simulink model "VCU_TDN"  (R2020a)
settings: Solver=FixedStepDiscrete  StartTime=0.0  StopTime=10.0  FixedStep=0.001  RelTol=1e-3  EnableMultiTasking=on
InitFcn:
  | EcoCoder_PreCheckLic();
undefined symbols (not defined in the file or in its folder): h, km
libraries: CoderSF_BSW_Libs x187, simulink x9, SF_CanService_Libs x1
(part 2 of 2)

== system VCU_TDN/Code/Initialization/Disabling the inverter ==
  Constant : Constant  Value=hex2dec('51')  OutDataTypeStr=uint8
  Constant1 : Constant  Value=hex2dec('0004')  OutDataTypeStr=uint16
  Pack Signals To CAN Data : CoderSF_BSW_Libs/CAN/Pack Signals To CAN Data  Signal="{{'REG_ID'  'Data1'},[0 8],[8 16],{'uint8'  'uint16'},{'Intel' 'Intel'}}"
  Send CAN Data : CoderSF_BSW_Libs/CAN/Send CAN Data  channel=CAN_A  txlen=3  txid=hex2dec('201')  frametype=Standard(11-bit ID)  showerror=off
  wires:
  Constant/1 -> Pack Signals To CAN Data/1
  Pack Signals To CAN Data/1 -> Send CAN Data/1
  Constant1/1 -> Pack Signals To CAN Data/2

== system VCU_TDN/Code/Ready to drive/Activate Ready to drive ==
  Trigger : TriggerPort  VariantControl=Variant
  Constant{,1,3..4} (4 alike) : Constant  OutDataTypeStr=boolean
  Enabling the inverter : Subsystem
  FRG/RUN : CoderSF_BSW_Libs/Digital I//O/Switch Output  channel=LSO07
  RFE : CoderSF_BSW_Libs/Digital I//O/Switch Output  channel=LSO06
  Ready to drive LED : CoderSF_BSW_Libs/Digital I//O/Switch Output  channel=LSO08
  Ready to drive sound : CoderSF_BSW_Libs/Digital I//O/Switch Output  channel=LSO10
  wires:
  Constant1/1 -> FRG/RUN/1
  Constant/1 -> RFE/1
  Constant3/1 -> Ready to drive LED/1
  Constant4/1 -> Ready to drive sound/1

== system VCU_TDN/Code/Ready to drive/Deactivate Ready to drive ==
  Trigger : TriggerPort  VariantControl=Variant
  Constant : Constant  Value=0  OutDataTypeStr=boolean
  Constant1 : Constant  Value=0  OutDataTypeStr=boolean
  Constant3 : Constant  Value=0  OutDataTypeStr=boolean
  Disabling the inverter : Subsystem
  FRG/RUN : CoderSF_BSW_Libs/Digital I//O/Switch Output  channel=LSO07
  RFE : CoderSF_BSW_Libs/Digital I//O/Switch Output  channel=LSO06
  Ready to drive LED : CoderSF_BSW_Libs/Digital I//O/Switch Output  channel=LSO08
  wires:
  Constant1/1 -> FRG/RUN/1
  Constant/1 -> RFE/1
  Constant3/1 -> Ready to drive LED/1

== system VCU_TDN/Code/Ready to drive/Stop RTD sound ==
  Trigger : TriggerPort  VariantControl=Variant
  Constant4 : Constant  Value=0  OutDataTypeStr=boolean
  Ready to drive sound : CoderSF_BSW_Libs/Digital I//O/Switch Output  channel=LSO10
  wires:
  Constant4/1 -> Ready to drive sound/1

== system VCU_TDN/Code/Receiving data/BMS ==

== system VCU_TDN/Code/Receiving data/Battery temperature sensors ==

== system VCU_TDN/Code/Receiving data/Inverter ==
  Data saving : Subsystem  TreatAsAtomicUnit=on
  Read CAN Message : SF_CanService_Libs/Read CAN Message  typeCAN=Connected  channel=CAN_A  mEn=off  msgInfo=can  msgIterm=INV_VCU  msgItermStore=INV_VCU  valid=on  stale=off  motoBit=off  setSignalName=off  flgCustomMonitorVariableRules=on  defineSignalName=off  prefixSignal='rx'  flgValTest=off  flgNoFixed=on  tSample=Task_L10ms  modeCode=Parameterless
  wires:
  Read CAN Message/1 -> Data saving/Trigger
  Read CAN Message/3 -> Data saving/2(Data)
  Read CAN Message/2 -> Data saving/1(RegID)

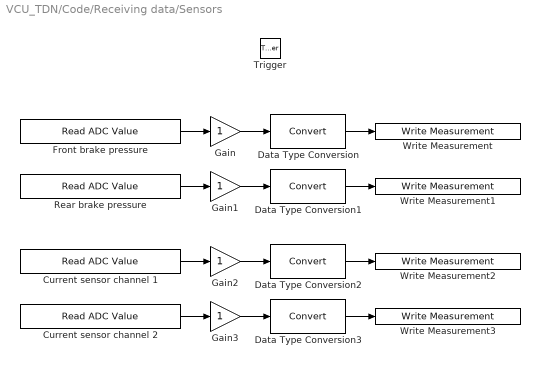
== system VCU_TDN/Code/Receiving data/Sensors ==
  Trigger : TriggerPort  TriggerType=function-call  VariantControl=Variant  PortDimensions=1
  Current sensor channel 1 : CoderSF_BSW_Libs/ADC/Read ADC Value  channel=15
  Current sensor channel 2 : CoderSF_BSW_Libs/ADC/Read ADC Value  channel=17
  Data Type Conversion{,1..3} (4 alike) : DataTypeConversion
  Front brake pressure : CoderSF_BSW_Libs/ADC/Read ADC Value  channel=8
  Gain{,1..3} (4 alike) : Gain
  Rear brake pressure : CoderSF_BSW_Libs/ADC/Read ADC Value  channel=12
  Write Measurement : CoderSF_BSW_Libs/Calibration & Measurement/Write Measurement  variable_name=FR_BRK_PRESSURE  variable_value=0  variable_type=single  numD=1  unitStr=bar  descStr=""
      settings: AttributesFormatString=type:%<variable_type> Dimensions:%<numD>
  Write Measurement1 : CoderSF_BSW_Libs/Calibration & Measurement/Write Measurement  variable_name=RR_BRAKE_PRESSURE  variable_value=0  variable_type=single  numD=1  unitStr=bar  descStr=""
      settings: AttributesFormatString=type:%<variable_type> Dimensions:%<numD>
  Write Measurement2 : CoderSF_BSW_Libs/Calibration & Measurement/Write Measurement  variable_name=CURRENT_CH_1  variable_value=0  variable_type=int16  numD=1  unitStr=A  descStr=""
      settings: AttributesFormatString=type:%<variable_type> Dimensions:%<numD>
  Write Measurement3 : CoderSF_BSW_Libs/Calibration & Measurement/Write Measurement  variable_name=CURRENT_CH_2  variable_value=0  variable_type=int16  numD=1  unitStr=A  descStr=""
      settings: AttributesFormatString=type:%<variable_type> Dimensions:%<numD>
  wires:
  Current sensor channel 2/1 -> Gain3/1
  Current sensor channel 1/1 -> Gain2/1
  Rear brake pressure/1 -> Gain1/1
  Front brake pressure/1 -> Gain/1
  Data Type Conversion/1 -> Write Measurement/1
  Data Type Conversion3/1 -> Write Measurement3/1
  Gain2/1 -> Data Type Conversion2/1
  Data Type Conversion2/1 -> Write Measurement2/1
  Gain1/1 -> Data Type Conversion1/1
  Data Type Conversion1/1 -> Write Measurement1/1
  Gain/1 -> Data Type Conversion/1
  Gain3/1 -> Data Type Conversion3/1

== system VCU_TDN/Code/Ready to drive/Activate Ready to drive/Enabling the inverter ==
  Constant : Constant  Value=hex2dec('51')  OutDataTypeStr=uint8
  Constant1 : Constant  Value=hex2dec('0000')  OutDataTypeStr=uint16
  Pack Signals To CAN Data : CoderSF_BSW_Libs/CAN/Pack Signals To CAN Data  Signal="{{'REG_ID'  'Data1'},[0 8],[8 16],{'uint8'  'uint16'},{'Intel' 'Intel'}}"
  Send CAN Data : CoderSF_BSW_Libs/CAN/Send CAN Data  channel=CAN_A  txlen=3  txid=hex2dec('201')  frametype=Standard(11-bit ID)  showerror=off
  wires:
  Constant/1 -> Pack Signals To CAN Data/1
  Pack Signals To CAN Data/1 -> Send CAN Data/1
  Constant1/1 -> Pack Signals To CAN Data/2

== system VCU_TDN/Code/Ready to drive/Deactivate Ready to drive/Disabling the inverter ==
  Constant : Constant  Value=hex2dec('51')  OutDataTypeStr=uint8
  Constant1 : Constant  Value=hex2dec('0004')  OutDataTypeStr=uint16
  Pack Signals To CAN Data : CoderSF_BSW_Libs/CAN/Pack Signals To CAN Data  Signal="{{'REG_ID'  'Data1'},[0 8],[8 16],{'uint8'  'uint16'},{'Intel' 'Intel'}}"
  Send CAN Data : CoderSF_BSW_Libs/CAN/Send CAN Data  channel=CAN_A  txlen=3  txid=hex2dec('201')  frametype=Standard(11-bit ID)  showerror=off
  wires:
  Constant/1 -> Pack Signals To CAN Data/1
  Pack Signals To CAN Data/1 -> Send CAN Data/1
  Constant1/1 -> Pack Signals To CAN Data/2

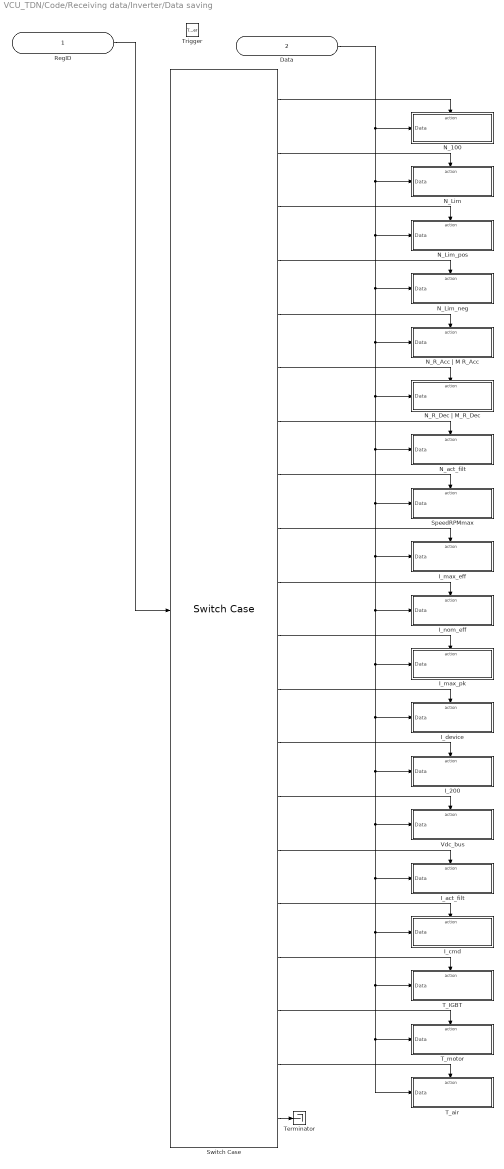
== system VCU_TDN/Code/Receiving data/Inverter/Data saving ==
  RegID : Inport
  Data : Inport  Port=2
  Trigger : TriggerPort  VariantControl=Variant
  I_200 : Subsystem  TreatAsAtomicUnit=on
  I_act_filt : Subsystem  TreatAsAtomicUnit=on
  I_cmd : Subsystem  TreatAsAtomicUnit=on
  I_device : Subsystem  TreatAsAtomicUnit=on
  I_max_eff : Subsystem  TreatAsAtomicUnit=on
  I_max_pk : Subsystem  TreatAsAtomicUnit=on
  I_nom_eff : Subsystem  TreatAsAtomicUnit=on
  N_100 : Subsystem  TreatAsAtomicUnit=on
  N_Lim : Subsystem  TreatAsAtomicUnit=on
  N_Lim_neg : Subsystem  TreatAsAtomicUnit=on
  N_Lim_pos : Subsystem  TreatAsAtomicUnit=on
  N_R_Acc | M R_Acc : Subsystem  TreatAsAtomicUnit=on
  N_R_Dec | M_R_Dec : Subsystem  TreatAsAtomicUnit=on
  N_act_filt : Subsystem  TreatAsAtomicUnit=on
  SpeedRPMmax : Subsystem  TreatAsAtomicUnit=on
  Switch Case : SwitchCase  CaseConditions={0xc8,0x34,0x3f,0x3e,0x35,0xed,0xce,0xa8,0x4d,0x4e,0xc4,0xc6,0xd9,0xeb,0x5f,0x26,0x4a,0x49,0x4b}
  T_IGBT : Subsystem  TreatAsAtomicUnit=on
  T_air : Subsystem  TreatAsAtomicUnit=on
  T_motor : Subsystem  TreatAsAtomicUnit=on
  Terminator : Terminator
  Vdc_bus : Subsystem  TreatAsAtomicUnit=on
  wires:
  RegID/1 -> Switch Case/1
  Switch Case/20 -> Terminator/1
  Switch Case/1 -> N_100/Action
  Switch Case/2 -> N_Lim/Action
  Switch Case/3 -> N_Lim_pos/Action
  Switch Case/4 -> N_Lim_neg/Action
  Switch Case/5 -> N_R_Acc | M R_Acc/Action
  Switch Case/6 -> N_R_Dec | M_R_Dec/Action
  Switch Case/7 -> N_act_filt/Action
  Switch Case/8 -> SpeedRPMmax/Action
  Switch Case/9 -> I_max_eff/Action
  Switch Case/10 -> I_nom_eff/Action
  Switch Case/11 -> I_max_pk/Action
  Switch Case/12 -> I_device/Action
  Switch Case/13 -> I_200/Action
  Switch Case/14 -> Vdc_bus/Action
  Switch Case/15 -> I_act_filt/Action
  Switch Case/16 -> I_cmd/Action
  Switch Case/17 -> T_IGBT/Action
  Switch Case/18 -> T_motor/Action
  Switch Case/19 -> T_air/Action
  Data/1 -> T_air/1(Data), T_motor/1(Data), T_IGBT/1(Data), I_cmd/1(Data), I_act_filt/1(Data), Vdc_bus/1(Data), I_200/1(Data), I_device/1(Data), I_max_pk/1(Data), I_nom_eff/1(Data), I_max_eff/1(Data), SpeedRPMmax/1(Data), N_act_filt/1(Data), N_R_Dec | M_R_Dec/1(Data), N_R_Acc | M R_Acc/1(Data), N_Lim_neg/1(Data), N_Lim_pos/1(Data), N_Lim/1(Data), N_100/1(Data)

== system VCU_TDN/Code/Receiving data/Inverter/Data saving/I_200 ==
  Data : Inport
  Action Port : ActionPort  ActionPortLabel=case [ 217 ]:
  Data Type Conversion : DataTypeConversion
  Write NVM : CoderSF_BSW_Libs/Non-volatile Memory Blocks/Write NVM  variable_name=nvmI_200  flgDef=on  variable_value=0  variable_type=int16  variable_numD=1  unitStr=""  descStr=""  EcoCoderBlockID=N001_NVMVDEF
      settings: AttributesFormatString=value:%<variable_value> type:%<variable_type> D:%<variable_numD>
  Write and Read Measurement : CoderSF_BSW_Libs/Calibration & Measurement/Write and Read Measurement  variable_name=I_200  variable_value=0  variable_type=int16  numD=1  unitStr=""  descStr=""
      settings: AttributesFormatString=type:%<variable_type> Dimensions:%<numD>
  wires:
  Data Type Conversion/1 -> Write and Read Measurement/1
  Data/1 -> Data Type Conversion/1
  Write and Read Measurement/1 -> Write NVM/1  "I_200"

== system VCU_TDN/Code/Receiving data/Inverter/Data saving/I_act_filt ==
  Data : Inport
  Action Port : ActionPort  ActionPortLabel=case [ 95 ]:
  Data Type Conversion : DataTypeConversion
  Write NVM : CoderSF_BSW_Libs/Non-volatile Memory Blocks/Write NVM  variable_name=nvmI_act_filt  flgDef=on  variable_value=0  variable_type=int16  variable_numD=1  unitStr=""  descStr=""  EcoCoderBlockID=N001_NVMVDEF
      settings: AttributesFormatString=value:%<variable_value> type:%<variable_type> D:%<variable_numD>
  Write and Read Measurement : CoderSF_BSW_Libs/Calibration & Measurement/Write and Read Measurement  variable_name=I_act_filt  variable_value=0  variable_type=int16  numD=1  unitStr=""  descStr=""
      settings: AttributesFormatString=type:%<variable_type> Dimensions:%<numD>
  wires:
  Data Type Conversion/1 -> Write and Read Measurement/1
  Data/1 -> Data Type Conversion/1
  Write and Read Measurement/1 -> Write NVM/1  "I_act_filt"

== system VCU_TDN/Code/Receiving data/Inverter/Data saving/I_cmd ==
  Data : Inport
  Action Port : ActionPort  ActionPortLabel=case [ 38 ]:
  Data Type Conversion : DataTypeConversion
  Write NVM : CoderSF_BSW_Libs/Non-volatile Memory Blocks/Write NVM  variable_name=nvmI_cmd  flgDef=on  variable_value=0  variable_type=int16  variable_numD=1  unitStr=""  descStr=""  EcoCoderBlockID=N001_NVMVDEF
      settings: AttributesFormatString=value:%<variable_value> type:%<variable_type> D:%<variable_numD>
  Write and Read Measurement : CoderSF_BSW_Libs/Calibration & Measurement/Write and Read Measurement  variable_name=I_cmd  variable_value=0  variable_type=int16  numD=1  unitStr=""  descStr=""
      settings: AttributesFormatString=type:%<variable_type> Dimensions:%<numD>
  wires:
  Data Type Conversion/1 -> Write and Read Measurement/1
  Data/1 -> Data Type Conversion/1
  Write and Read Measurement/1 -> Write NVM/1  "I_cmd"

== system VCU_TDN/Code/Receiving data/Inverter/Data saving/I_device ==
  Data : Inport
  Action Port : ActionPort  ActionPortLabel=case [ 198 ]:
  Data Type Conversion : DataTypeConversion
  Write NVM : CoderSF_BSW_Libs/Non-volatile Memory Blocks/Write NVM  variable_name=nvmI_device  flgDef=on  variable_value=0  variable_type=int16  variable_numD=1  unitStr=""  descStr=""  EcoCoderBlockID=N001_NVMVDEF
      settings: AttributesFormatString=value:%<variable_value> type:%<variable_type> D:%<variable_numD>
  Write and Read Measurement : CoderSF_BSW_Libs/Calibration & Measurement/Write and Read Measurement  variable_name=I_device  variable_value=0  variable_type=int16  numD=1  unitStr=""  descStr=""
      settings: AttributesFormatString=type:%<variable_type> Dimensions:%<numD>
  wires:
  Data Type Conversion/1 -> Write and Read Measurement/1
  Data/1 -> Data Type Conversion/1
  Write and Read Measurement/1 -> Write NVM/1  "I_device"

== system VCU_TDN/Code/Receiving data/Inverter/Data saving/I_max_eff ==
  Data : Inport
  Action Port : ActionPort  ActionPortLabel=case [ 77 ]:
  Data Type Conversion : DataTypeConversion
  Write NVM : CoderSF_BSW_Libs/Non-volatile Memory Blocks/Write NVM  variable_name=nvmI_max_eff  flgDef=on  variable_value=0  variable_type=int16  variable_numD=1  unitStr=""  descStr=""  EcoCoderBlockID=N001_NVMVDEF
      settings: AttributesFormatString=value:%<variable_value> type:%<variable_type> D:%<variable_numD>
  Write and Read Measurement : CoderSF_BSW_Libs/Calibration & Measurement/Write and Read Measurement  variable_name=I_max_eff  variable_value=0  variable_type=int16  numD=1  unitStr=""  descStr=""
      settings: AttributesFormatString=type:%<variable_type> Dimensions:%<numD>
  wires:
  Data Type Conversion/1 -> Write and Read Measurement/1
  Data/1 -> Data Type Conversion/1
  Write and Read Measurement/1 -> Write NVM/1  "I_max_eff"

== system VCU_TDN/Code/Receiving data/Inverter/Data saving/I_max_pk ==
  Data : Inport
  Action Port : ActionPort  ActionPortLabel=case [ 196 ]:
  Data Type Conversion : DataTypeConversion
  Write NVM : CoderSF_BSW_Libs/Non-volatile Memory Blocks/Write NVM  variable_name=nvmI_max_pk  flgDef=on  variable_value=0  variable_type=int16  variable_numD=1  unitStr=""  descStr=""  EcoCoderBlockID=N001_NVMVDEF
      settings: AttributesFormatString=value:%<variable_value> type:%<variable_type> D:%<variable_numD>
  Write and Read Measurement : CoderSF_BSW_Libs/Calibration & Measurement/Write and Read Measurement  variable_name=I_max_pk  variable_value=0  variable_type=int16  numD=1  unitStr=""  descStr=""
      settings: AttributesFormatString=type:%<variable_type> Dimensions:%<numD>
  wires:
  Data Type Conversion/1 -> Write and Read Measurement/1
  Data/1 -> Data Type Conversion/1
  Write and Read Measurement/1 -> Write NVM/1  "I_max_pk"

== system VCU_TDN/Code/Receiving data/Inverter/Data saving/I_nom_eff ==
  Data : Inport
  Action Port : ActionPort  ActionPortLabel=case [ 78 ]:
  Data Type Conversion : DataTypeConversion
  Write NVM : CoderSF_BSW_Libs/Non-volatile Memory Blocks/Write NVM  variable_name=nvmI_nom_eff  flgDef=on  variable_value=0  variable_type=int16  variable_numD=1  unitStr=""  descStr=""  EcoCoderBlockID=N001_NVMVDEF
      settings: AttributesFormatString=value:%<variable_value> type:%<variable_type> D:%<variable_numD>
  Write and Read Measurement : CoderSF_BSW_Libs/Calibration & Measurement/Write and Read Measurement  variable_name=I_nom_eff  variable_value=0  variable_type=int16  numD=1  unitStr=""  descStr=""
      settings: AttributesFormatString=type:%<variable_type> Dimensions:%<numD>
  wires:
  Data Type Conversion/1 -> Write and Read Measurement/1
  Data/1 -> Data Type Conversion/1
  Write and Read Measurement/1 -> Write NVM/1  "I_nom_eff"

== system VCU_TDN/Code/Receiving data/Inverter/Data saving/N_100 ==
  Data : Inport
  Action Port : ActionPort  ActionPortLabel=case [ 200 ]:
  Data Type Conversion : DataTypeConversion
  Write NVM : CoderSF_BSW_Libs/Non-volatile Memory Blocks/Write NVM  variable_name=nvmN_100  flgDef=on  variable_value=0  variable_type=uint16  variable_numD=1  unitStr=""  descStr=""  EcoCoderBlockID=N001_NVMVDEF
      settings: AttributesFormatString=value:%<variable_value> type:%<variable_type> D:%<variable_numD>
  Write and Read Measurement : CoderSF_BSW_Libs/Calibration & Measurement/Write and Read Measurement  variable_name=N_100  variable_value=0  variable_type=uint16  numD=1  unitStr=""  descStr=""
      settings: AttributesFormatString=type:%<variable_type> Dimensions:%<numD>
  wires:
  Data Type Conversion/1 -> Write and Read Measurement/1
  Data/1 -> Data Type Conversion/1
  Write and Read Measurement/1 -> Write NVM/1  "N_100"

== system VCU_TDN/Code/Receiving data/Inverter/Data saving/N_Lim ==
  Data : Inport
  Action Port : ActionPort  ActionPortLabel=case [ 52 ]:
  Data Type Conversion : DataTypeConversion
  Write NVM : CoderSF_BSW_Libs/Non-volatile Memory Blocks/Write NVM  variable_name=nvmN_lim  flgDef=on  variable_value=0  variable_type=uint16  variable_numD=1  unitStr=""  descStr=""  EcoCoderBlockID=N001_NVMVDEF
      settings: AttributesFormatString=value:%<variable_value> type:%<variable_type> D:%<variable_numD>
  Write and Read Measurement : CoderSF_BSW_Libs/Calibration & Measurement/Write and Read Measurement  variable_name=N_lim  variable_value=0  variable_type=uint16  numD=1  unitStr=""  descStr=""
      settings: AttributesFormatString=type:%<variable_type> Dimensions:%<numD>
  wires:
  Data Type Conversion/1 -> Write and Read Measurement/1
  Data/1 -> Data Type Conversion/1
  Write and Read Measurement/1 -> Write NVM/1  "N_lim"

== system VCU_TDN/Code/Receiving data/Inverter/Data saving/N_Lim_neg ==
  Data : Inport
  Action Port : ActionPort  ActionPortLabel=case [ 62 ]:
  Data Type Conversion : DataTypeConversion
  Write NVM : CoderSF_BSW_Libs/Non-volatile Memory Blocks/Write NVM  variable_name=nvmN_lim_neg  flgDef=on  variable_value=0  variable_type=int16  variable_numD=1  unitStr=""  descStr=""  EcoCoderBlockID=N001_NVMVDEF
      settings: AttributesFormatString=value:%<variable_value> type:%<variable_type> D:%<variable_numD>
  Write and Read Measurement : CoderSF_BSW_Libs/Calibration & Measurement/Write and Read Measurement  variable_name=N_lim_neg  variable_value=0  variable_type=int16  numD=1  unitStr=""  descStr=""
      settings: AttributesFormatString=type:%<variable_type> Dimensions:%<numD>
  wires:
  Data Type Conversion/1 -> Write and Read Measurement/1
  Data/1 -> Data Type Conversion/1
  Write and Read Measurement/1 -> Write NVM/1  "N_lim_neg"

== system VCU_TDN/Code/Receiving data/Inverter/Data saving/N_Lim_pos ==
  Data : Inport
  Action Port : ActionPort  ActionPortLabel=case [ 63 ]:
  Data Type Conversion : DataTypeConversion
  Write NVM : CoderSF_BSW_Libs/Non-volatile Memory Blocks/Write NVM  variable_name=nvmN_lim_pos  flgDef=on  variable_value=0  variable_type=int16  variable_numD=1  unitStr=""  descStr=""  EcoCoderBlockID=N001_NVMVDEF
      settings: AttributesFormatString=value:%<variable_value> type:%<variable_type> D:%<variable_numD>
  Write and Read Measurement : CoderSF_BSW_Libs/Calibration & Measurement/Write and Read Measurement  variable_name=N_lim_pos  variable_value=0  variable_type=int16  numD=1  unitStr=""  descStr=""
      settings: AttributesFormatString=type:%<variable_type> Dimensions:%<numD>
  wires:
  Data Type Conversion/1 -> Write and Read Measurement/1
  Data/1 -> Data Type Conversion/1
  Write and Read Measurement/1 -> Write NVM/1  "N_lim_pos"

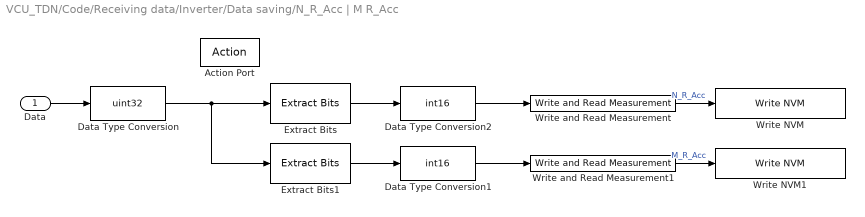
== system VCU_TDN/Code/Receiving data/Inverter/Data saving/N_R_Acc | M R_Acc ==
  Data : Inport
  Action Port : ActionPort  ActionPortLabel=case [ 53 ]:
  Data Type Conversion : DataTypeConversion  OutDataTypeStr=uint32
  Data Type Conversion1 : DataTypeConversion  OutDataTypeStr=int16
  Data Type Conversion2 : DataTypeConversion  OutDataTypeStr=int16
  Extract Bits : simulink/Logic and Bit Operations/Extract Bits  bitsToExtract=Lower half  numBits=8  bitIdxRange=[0 7]  outScalingMode=Treat bit field as an integer
  Extract Bits1 : simulink/Logic and Bit Operations/Extract Bits  bitsToExtract=Upper half  numBits=8  bitIdxRange=[0 7]  outScalingMode=Treat bit field as an integer
  Write NVM : CoderSF_BSW_Libs/Non-volatile Memory Blocks/Write NVM  variable_name=nvmN_R_Acc  flgDef=on  variable_value=0  variable_type=int16  variable_numD=1  unitStr=""  descStr=""  EcoCoderBlockID=N001_NVMVDEF
      settings: AttributesFormatString=value:%<variable_value> type:%<variable_type> D:%<variable_numD>
  Write NVM1 : CoderSF_BSW_Libs/Non-volatile Memory Blocks/Write NVM  variable_name=nvmM_R_Acc  flgDef=on  variable_value=0  variable_type=int16  variable_numD=1  unitStr=""  descStr=""  EcoCoderBlockID=N001_NVMVDEF
      settings: AttributesFormatString=value:%<variable_value> type:%<variable_type> D:%<variable_numD>
  Write and Read Measurement : CoderSF_BSW_Libs/Calibration & Measurement/Write and Read Measurement  variable_name=N_R_Acc  variable_value=0  variable_type=int16  numD=1  unitStr=""  descStr=""
      settings: AttributesFormatString=type:%<variable_type> Dimensions:%<numD>
  Write and Read Measurement1 : CoderSF_BSW_Libs/Calibration & Measurement/Write and Read Measurement  variable_name=M_R_Acc  variable_value=0  variable_type=int16  numD=1  unitStr=""  descStr=""
      settings: AttributesFormatString=type:%<variable_type> Dimensions:%<numD>
  wires:
  Data/1 -> Data Type Conversion/1
  Data Type Conversion/1 -> Extract Bits1/1, Extract Bits/1
  Extract Bits/1 -> Data Type Conversion2/1
  Data Type Conversion2/1 -> Write and Read Measurement/1
  Extract Bits1/1 -> Data Type Conversion1/1
  Data Type Conversion1/1 -> Write and Read Measurement1/1
  Write and Read Measurement/1 -> Write NVM/1  "N_R_Acc"
  Write and Read Measurement1/1 -> Write NVM1/1  "M_R_Acc"

== system VCU_TDN/Code/Receiving data/Inverter/Data saving/N_R_Dec | M_R_Dec ==
  Data : Inport
  Action Port : ActionPort  ActionPortLabel=case [ 237 ]:
  Data Type Conversion : DataTypeConversion  OutDataTypeStr=uint32
  Data Type Conversion1 : DataTypeConversion  OutDataTypeStr=int16
  Data Type Conversion2 : DataTypeConversion  OutDataTypeStr=int16
  Extract Bits : simulink/Logic and Bit Operations/Extract Bits  bitsToExtract=Lower half  numBits=8  bitIdxRange=[0 7]  outScalingMode=Treat bit field as an integer
  Extract Bits1 : simulink/Logic and Bit Operations/Extract Bits  bitsToExtract=Upper half  numBits=8  bitIdxRange=[0 7]  outScalingMode=Treat bit field as an integer
  Write NVM : CoderSF_BSW_Libs/Non-volatile Memory Blocks/Write NVM  variable_name=nvmN_R_Dec  flgDef=on  variable_value=0  variable_type=int16  variable_numD=1  unitStr=""  descStr=""  EcoCoderBlockID=N001_NVMVDEF
      settings: AttributesFormatString=value:%<variable_value> type:%<variable_type> D:%<variable_numD>
  Write NVM1 : CoderSF_BSW_Libs/Non-volatile Memory Blocks/Write NVM  variable_name=nvmM_R_Dec  flgDef=on  variable_value=0  variable_type=int16  variable_numD=1  unitStr=""  descStr=""  EcoCoderBlockID=N001_NVMVDEF
      settings: AttributesFormatString=value:%<variable_value> type:%<variable_type> D:%<variable_numD>
  Write and Read Measurement : CoderSF_BSW_Libs/Calibration & Measurement/Write and Read Measurement  variable_name=N_R_Dec  variable_value=0  variable_type=int16  numD=1  unitStr=""  descStr=""
      settings: AttributesFormatString=type:%<variable_type> Dimensions:%<numD>
  Write and Read Measurement1 : CoderSF_BSW_Libs/Calibration & Measurement/Write and Read Measurement  variable_name=M_R_Dec  variable_value=0  variable_type=int16  numD=1  unitStr=""  descStr=""
      settings: AttributesFormatString=type:%<variable_type> Dimensions:%<numD>
  wires:
  Data/1 -> Data Type Conversion/1
  Data Type Conversion2/1 -> Write and Read Measurement/1
  Data Type Conversion1/1 -> Write and Read Measurement1/1
  Data Type Conversion/1 -> Extract Bits1/1, Extract Bits/1
  Extract Bits1/1 -> Data Type Conversion1/1
  Extract Bits/1 -> Data Type Conversion2/1
  Write and Read Measurement/1 -> Write NVM/1  "N_R_Dec"
  Write and Read Measurement1/1 -> Write NVM1/1  "M_R_Dec"

== system VCU_TDN/Code/Receiving data/Inverter/Data saving/N_act_filt ==
  Data : Inport
  Action Port : ActionPort  ActionPortLabel=case [ 206 ]:
  Data Type Conversion : DataTypeConversion
  Write NVM : CoderSF_BSW_Libs/Non-volatile Memory Blocks/Write NVM  variable_name=nvmN_act_filt  flgDef=on  variable_value=0  variable_type=int16  variable_numD=1  unitStr=""  descStr=""  EcoCoderBlockID=N001_NVMVDEF
      settings: AttributesFormatString=value:%<variable_value> type:%<variable_type> D:%<variable_numD>
  Write and Read Measurement : CoderSF_BSW_Libs/Calibration & Measurement/Write and Read Measurement  variable_name=N_act_filt  variable_value=0  variable_type=int16  numD=1  unitStr=""  descStr=""
      settings: AttributesFormatString=type:%<variable_type> Dimensions:%<numD>
  wires:
  Data Type Conversion/1 -> Write and Read Measurement/1
  Data/1 -> Data Type Conversion/1
  Write and Read Measurement/1 -> Write NVM/1  "N_act_filt"

== system VCU_TDN/Code/Receiving data/Inverter/Data saving/SpeedRPMmax ==
  Data : Inport
  Action Port : ActionPort  ActionPortLabel=case [ 168 ]:
  Data Type Conversion : DataTypeConversion
  Write NVM : CoderSF_BSW_Libs/Non-volatile Memory Blocks/Write NVM  variable_name=nvmSpeedRPMmax  flgDef=on  variable_value=0  variable_type=int16  variable_numD=1  unitStr=""  descStr=""  EcoCoderBlockID=N001_NVMVDEF
      settings: AttributesFormatString=value:%<variable_value> type:%<variable_type> D:%<variable_numD>
  Write and Read Measurement : CoderSF_BSW_Libs/Calibration & Measurement/Write and Read Measurement  variable_name=SpeedRPMmax  variable_value=0  variable_type=int16  numD=1  unitStr=""  descStr=""
      settings: AttributesFormatString=type:%<variable_type> Dimensions:%<numD>
  wires:
  Data Type Conversion/1 -> Write and Read Measurement/1
  Data/1 -> Data Type Conversion/1
  Write and Read Measurement/1 -> Write NVM/1  "SpeedRPMmax"

== system VCU_TDN/Code/Receiving data/Inverter/Data saving/T_IGBT ==
  Data : Inport
  Action Port : ActionPort  ActionPortLabel=case [ 74 ]:
  Data Type Conversion : DataTypeConversion
  Write NVM : CoderSF_BSW_Libs/Non-volatile Memory Blocks/Write NVM  variable_name=nvmT_IGBT  flgDef=on  variable_value=0  variable_type=int16  variable_numD=1  unitStr=""  descStr=""  EcoCoderBlockID=N001_NVMVDEF
      settings: AttributesFormatString=value:%<variable_value> type:%<variable_type> D:%<variable_numD>
  Write and Read Measurement : CoderSF_BSW_Libs/Calibration & Measurement/Write and Read Measurement  variable_name=T_IGBT  variable_value=0  variable_type=int16  numD=1  unitStr=""  descStr=""
      settings: AttributesFormatString=type:%<variable_type> Dimensions:%<numD>
  wires:
  Data Type Conversion/1 -> Write and Read Measurement/1
  Data/1 -> Data Type Conversion/1
  Write and Read Measurement/1 -> Write NVM/1  "T_IGBT"

== system VCU_TDN/Code/Receiving data/Inverter/Data saving/T_air ==
  Data : Inport
  Action Port : ActionPort  ActionPortLabel=case [ 75 ]:
  Data Type Conversion : DataTypeConversion
  Write NVM : CoderSF_BSW_Libs/Non-volatile Memory Blocks/Write NVM  variable_name=nvmT_air  flgDef=on  variable_value=0  variable_type=int16  variable_numD=1  unitStr=""  descStr=""  EcoCoderBlockID=N001_NVMVDEF
      settings: AttributesFormatString=value:%<variable_value> type:%<variable_type> D:%<variable_numD>
  Write and Read Measurement : CoderSF_BSW_Libs/Calibration & Measurement/Write and Read Measurement  variable_name=T_air  variable_value=0  variable_type=int16  numD=1  unitStr=""  descStr=""
      settings: AttributesFormatString=type:%<variable_type> Dimensions:%<numD>
  wires:
  Data Type Conversion/1 -> Write and Read Measurement/1
  Data/1 -> Data Type Conversion/1
  Write and Read Measurement/1 -> Write NVM/1  "T_air"

== system VCU_TDN/Code/Receiving data/Inverter/Data saving/T_motor ==
  Data : Inport
  Action Port : ActionPort  ActionPortLabel=case [ 73 ]:
  Data Type Conversion : DataTypeConversion
  Write NVM : CoderSF_BSW_Libs/Non-volatile Memory Blocks/Write NVM  variable_name=nvmT_motor  flgDef=on  variable_value=0  variable_type=int16  variable_numD=1  unitStr=""  descStr=""  EcoCoderBlockID=N001_NVMVDEF
      settings: AttributesFormatString=value:%<variable_value> type:%<variable_type> D:%<variable_numD>
  Write and Read Measurement : CoderSF_BSW_Libs/Calibration & Measurement/Write and Read Measurement  variable_name=T_motor  variable_value=0  variable_type=int16  numD=1  unitStr=""  descStr=""
      settings: AttributesFormatString=type:%<variable_type> Dimensions:%<numD>
  wires:
  Data Type Conversion/1 -> Write and Read Measurement/1
  Data/1 -> Data Type Conversion/1
  Write and Read Measurement/1 -> Write NVM/1  "T_motor"

== system VCU_TDN/Code/Receiving data/Inverter/Data saving/Vdc_bus ==
  Data : Inport
  Action Port : ActionPort  ActionPortLabel=case [ 235 ]:
  Data Type Conversion : DataTypeConversion
  Write NVM : CoderSF_BSW_Libs/Non-volatile Memory Blocks/Write NVM  variable_name=nvmVdc_bus  flgDef=on  variable_value=0  variable_type=int16  variable_numD=1  unitStr=""  descStr=""  EcoCoderBlockID=N001_NVMVDEF
      settings: AttributesFormatString=value:%<variable_value> type:%<variable_type> D:%<variable_numD>
  Write and Read Measurement : CoderSF_BSW_Libs/Calibration & Measurement/Write and Read Measurement  variable_name=Vdc_bus  variable_value=0  variable_type=int16  numD=1  unitStr=""  descStr=""
      settings: AttributesFormatString=type:%<variable_type> Dimensions:%<numD>
  wires:
  Data Type Conversion/1 -> Write and Read Measurement/1
  Data/1 -> Data Type Conversion/1
  Write and Read Measurement/1 -> Write NVM/1  "Vdc_bus"
